simulink library "SimFly_Sensors"  (R2015b)
settings: Solver=VariableStepAuto  StartTime=0.0  StopTime=10.0  RelTol=1e-3
(part 2 of 2)

== matlab function SimFly_Sensors/GPS_UBX ==
  settings: updateMethod=DISCRETE  sampleTime=ubx_sample_time
  data: Ts output; lla output; flag_lla output; vel output; flag_vel output; sat output; alive output; time_delta output
function [Ts,lla,flag_lla,vel,flag_vel,sat,alive,time_delta] = ubx()
% Simulink Arduino Block Driver Library for Autocode Generation
 % 
 % This file is part of the Simulink Arduino Block Driver Library 
 % for Autocode Generation with Simulink
 %
 % This Library is free software: you can redistribute it and/or modify
 % it under the terms of the GNU General Public License as published by
 % the Free Software Foundation, either version 3 of the License, or
 % (at your option) any later version.
 %
 % This Library is distributed in the hope that it will be useful,
 % but WITHOUT ANY WARRANTY; without even the implied warranty of
 % MERCHANTABILITY or FITNESS FOR A PARTICULAR PURPOSE.  See the
 % GNU General Public License for more details.
 %
 % You should have received a copy of the GNU General Public License
 % along with this Library.  If not, see
 % <http://www.gnu.org/licenses/>.
 %
%
%PURPOSE: Driver for GPS UBX with hardware abstraction layer
%AUTHOR: Marcell Mocher
%DATE: 16.6.2016
%VERSION: 0.1 V Fist build
%Input: -
%Output:    Ts[1](uint32) =  GPS Millisecond from read
%           lla[3,1](double) =  Longitude Latitude Altitude in [deg] alt in [m]
%           flag_lla(boolean) = boolean for lla update 5Hz
%           vel[3,1](single) = ECEF X Y Z velocity m/s
%           flag_vel(boolean) = boolean for velocity update 5Hz
%           sat[1](uint8) = Number of visible satalites
%           alive[1](boolean) = Flag if UPX is alive and reads signals
%           with 5Hz update rate
%           time_delta(single) = time needed to execute funtion [us]
%Info: This drive requires function call triggered simuluink functions in
% order to work
%Requires:  [double] = getTime(),
%           [val_read] =  ardu_Serial1(uint8(called_function),uint32(baudrate),uint8(write_value));

persistent init_flag alive_flag state ck1 ck2 code id length idx data chk1...
    chk2 lastTime ack_count ack_flag lon lat alt gps_flag ecefXv ecefYv...
    ecefZv numSV vel_flag gps_num vel_num

if strcmp(coder.target, 'rtw'),
    
    
time_start = uint32(0);
time_start = coder.ceval('_get_time');

% Parameter from Mask!
baud = uint32(38400); % Standard Baudrate for UBX

% Init parameters

if isempty(init_flag)
    init_flag = 0;
    alive_flag = true;
    
    state = uint8(0);
    ck1 = uint64(0);
    ck2 = uint64(0);
    code = uint8(0);
    id = uint8(0);
    length = uint16(0);
    idx = uint16(0);
    data = uint8(zeros(512,1));
    chk1 = uint8(0);
    chk2 = uint8(0);
    lastTime = uint32(0);
    
    lon = double(0);
    lat = double(0);
    alt = double(0);
    ecefXv = single(0);
    ecefYv = single(0);
    ecefZv = single(0);
    numSV  = uint8(0);
    gps_num = uint8(0);
    vel_num = uint8(0);
    
    %Init Serial1 at 38000 baud
    coder.ceval('_serial_init',uint8(1),baud);
    
    ack_size= uint16(1); % Enter num of commands send!
    ack_flag = uint16(zeros(ack_size,1)); % Enter num of commands send!
    ack_count = uint16(1);
    
end

gps_flag = false;
vel_flag = false;

cc = uint8(0);
av = uint8(0);
av = coder.ceval('_serial_available',uint8(1));
if av > 0
    for i = 1:20
        cc = coder.ceval('_serial_read',uint8(1));
        switch state
            case 0 %wait for sync 1 (0xB5)
                ck1 = uint64(0);
                ck2 = uint64(0);
                if cc == 181 %0xB5
                    state = state + 1;
                end
            case 1 %wait for sync 2 (0x62)
                if cc == 98
                    state = state + 1;
                else
                    state = uint8(0);
                end
            case 2 %wait for class code
                code = cc;
                ck1 = ck1 + uint64(cc);
                if ck1 >= 256
                    ck1 = ck1 - uint64(256);
                end
                ck2 = ck2 + ck1;
                if ck2 >= 256
                    ck2 = ck2 - uint64(256);
                end
                state = state +1;
            case 3    % wait for Id
                id = cc;
                ck1 = ck1 + uint64(cc);
                if ck1 >= 256
                    ck1 = ck1 - uint64(256);
                end
                ck2 = ck2 + ck1;
                if ck2 >= 256
                    ck2 = ck2 - uint64(256);
                end
                state = state +1;
            case 4    % wait for length byte 1
                length = uint16(cc);
                ck1 = ck1 + uint64(cc);
                if ck1 >= 256
                    ck1 = ck1 - uint64(256);
                end
                ck2 = ck2 + ck1;
                if ck2 >= 256
                    ck2 = ck2 - uint64(256);
                end
                state = state +1;
            case 5   % wait for length byte 2
                val = uint16(cc);
                length = bitor(bitshift(val,8),length);
                ck1 = ck1 + uint64(cc);
                if ck1 >= 256
                    ck1 = ck1 - uint64(256);
                end
                ck2 = ck2 + ck1;
                if ck2 >= 256
                    ck2 = ck2 - uint64(256);
                end
                state = state + 1;
                idx = uint16(1);
                if length > 512
                    state = uint8(0);
                end
            case 6   % wait for <length> payload bytes
                data(idx) = cc;
                idx = idx + 1;
                ck1 = ck1 + uint64(cc);
                if ck1 >= 256
                    ck1 = ck1 - uint64(256);
                end
                ck2 = ck2 + ck1;
                if ck2 >= 256
                    ck2 = ck2 - uint64(256);
                end
                if (idx - 1 >= length)
                    state = state + 1;
                end
            case 7    % wait for checksum 1
                chk1 = cc;
                state = state + 1;
            case 8
                chk2 = cc;
                if (ck1 == chk1) && (ck2 == chk2)
                    switch code
                        case 1 %NAV-
                            lastTime = typecast(data(1:4),'uint32');
                            switch id
                                case 2 %NAV-POSLLH
                                    lon = double(typecast(data(5:8),'int32')) * 1e-7;
                                    lat = double(typecast(data(9:12),'int32')) * 1e-7;
                                    alt = double(typecast(data(13:16),'int32')) * 1e-3;
                                    gps_flag = true;
                                case 6 %NAV-SOL
                                    ecefXv = single(typecast(data(29:32),'int32')) * 1e-2; % m/s ECEF X velocity
                                    ecefYv = single(typecast(data(33:36),'int32')) * 1e-2; % m/s ECEF Y velocity
                                    ecefZv = single(typecast(data(37:40),'int32')) * 1e-2; % m/s ECEF Z velocity
                                    numSV  = typecast(data(48),'uint8'); % numSV
                                    vel_flag = true;
                            end
                        case 5 % ACK
                            switch id
                                case 0 % ACK-NAK Message Not Acknowledged
                                    if ack_count >= numel(ack_flag)
                                        ack_flag(ack_count) = false;
                                        ack_count = ack_count + 1;
                                    end
                                case 1 % ACK-NAK Message Acknowledged
                                    if ack_count >= numel(ack_flag)
                                        ack_flag(ack_count) = true;
                                        ack_count = ack_count + 1;
                                    end
                            end
                    end % End of switch (code)
                    state = uint8(0);
                else
                    state = uint8(0);
                end % End of checksum check
                
        end % End of switch (state)
        
    end % End for
    
end % End if

Ts = lastTime;
lla = [lon lat alt];
vel = [ecefXv ecefYv ecefZv];
sat = numSV;
flag_lla = gps_flag;
flag_vel = vel_flag;

if gps_flag == 0
    gps_num = gps_num + 1;
    if gps_num > 20
        alive_flag = false;
    end
else
    gps_num = uint8(0);
end

if vel_flag == 0
    vel_num = vel_num + 1;
    if vel_num > 20
        alive_flag = false;
    end
else
    vel_num = uint8(0);
end



% Only do readings if sensor is healthy
% if alive_flag == true
%
% end
alive = alive_flag;  %alive_flag;
time_end = uint32(0);
time_end = coder.ceval('_get_time');
time_delta = time_end - time_start;

else
Ts =  uint32(0);
lla = [0 0 0];
flag_lla = true;
vel = single([0 0 0]);
flag_vel = true;
sat = uint8(0);
alive = true;  %alive_flag;
time_delta = uint32(0);
end
end

== matlab function SimFly_Sensors/baro_alt ==
  settings: updateMethod=DISCRETE  sampleTime=alt_sample_time
  data: p input; baro_alt output; p0 parameter
function baro_alt  = baro_alt(p, p0)
% Simulink Arduino Block Driver Library for Autocode Generation
 % 
 % This file is part of the Simulink Arduino Block Driver Library 
 % for Autocode Generation with Simulink
 %
 % This Library is free software: you can redistribute it and/or modify
 % it under the terms of the GNU General Public License as published by
 % the Free Software Foundation, either version 3 of the License, or
 % (at your option) any later version.
 %
 % This Library is distributed in the hope that it will be useful,
 % but WITHOUT ANY WARRANTY; without even the implied warranty of
 % MERCHANTABILITY or FITNESS FOR A PARTICULAR PURPOSE.  See the
 % GNU General Public License for more details.
 %
 % You should have received a copy of the GNU General Public License
 % along with this Library.  If not, see
 % <http://www.gnu.org/licenses/>.
 %
%
%PURPOSE: Function to calculate the altitude from the pressure
%AUTHOR: Marcell Mocher
%DATE: 25.6.2016
%VERSION: 0.1 V Fist build
%Input: -
%Output:    alt[1](single) =  barometric altitude
%Info: 
%Requires:

%p0 = 1013.25;   % pressure at sea level in hPa

baro_alt = 44300*(1-(p/p0)^0.19); % barometric formula

== matlab function SimFly_Sensors/Gyro_L3GD20H ==
  settings: updateMethod=DISCRETE  sampleTime=l3gd20_sampletime
  data: gyro output; alive output; time_delta output; sD0Pin parameter; scaleValue parameter; freqValue parameter
function [gyro,alive,time_delta] = fcn(sD0Pin, scaleValue, freqValue)
% Simulink Arduino Block Driver Library for Autocode Generation
 % 
 % This file is part of the Simulink Arduino Block Driver Library 
 % for Autocode Generation with Simulink
 %
 % This Library is free software: you can redistribute it and/or modify
 % it under the terms of the GNU General Public License as published by
 % the Free Software Foundation, either version 3 of the License, or
 % (at your option) any later version.
 %
 % This Library is distributed in the hope that it will be useful,
 % but WITHOUT ANY WARRANTY; without even the implied warranty of
 % MERCHANTABILITY or FITNESS FOR A PARTICULAR PURPOSE.  See the
 % GNU General Public License for more details.
 %
 % You should have received a copy of the GNU General Public License
 % along with this Library.  If not, see
 % <http://www.gnu.org/licenses/>.
 %
%
%PURMPOSE: Driver for L3GD20H with hardware abstraction layer
%AUTHOR: Marcell Mocher
%DATE: 11.6.2016
%VERSION: 0.1V Fist build
%Input: -
%Output:    accel[3*1](single) = acceleration in X,Y,Z Axis [ms^-2]
%           mag[3*1](single) = magnetic field in X,Y,Z Axis [gauss]
%           alive(boolean) = boolean if sensor is alive
%           time_delta(single) = time needed to execute funtion [us]
%Info: This driver requires function call triggered simulink functions in
% order to work see requires
%Requires:  _get_time
%           _serial_init
%           _serial_print
%           _serial_write
%           _i2c_write_register
%           _i2c_read_register


persistent init_flag alive_flag sensibility L3GD20H_ADDR L3GD20_WHO_AM_I...
    L3GD20H_ID L3GD20_CTRL_REG1 L3GD20_CTRL_REG4

if strcmp(coder.target, 'rtw'),
    
    
    time_start = uint32(0);
    time_start = coder.ceval('_get_time');
    
    %Parameter from Mask!
    sd0 = sD0Pin;
    scale = scaleValue;
    freq = freqValue;
    
    if isempty(init_flag)
        init_flag = 0;
        alive_flag = false;
        gyro = single(zeros(3,1));
        L3GD20_WHO_AM_I = uint8(hex2dec('0F')); % Who AM I Register
        L3GD20H_ID = uint8(hex2dec('D7'));
        L3GD20_CTRL_REG1 = uint8(hex2dec('20'));
        L3GD20_CTRL_REG4 = uint8(hex2dec('23'));
        
        % Init functions
        coder.ceval('_i2c_init');
        
        % Assign MPU SA0 status
        if sd0 == true
            L3GD20H_ADDR = uint8(hex2dec('6B')); % High Address
        else
            L3GD20H_ADDR = uint8(hex2dec('6A')); % Low Address
        end
        
        %Check if sensor is connected
        val = uint8(zeros(6,1));
        coder.ceval('_i2c_read_register',L3GD20H_ADDR,L3GD20_WHO_AM_I,uint8(1),coder.ref(val));
        if  val(1) == L3GD20H_ID
            alive_flag = true;
        end
        
        % Start with normal mode -> all axes enabled
        % Datasheet = p36
        % Register 0x0F = 100Hz 12.5 Cutt of Hz
        % Register 0x1F = 100Hz 25 Cutt of Hz
        % Register 0x5F = 200Hz 0 Cutt of Hz
        % Register 0x4F = 200Hz 12.5 Cutt of Hz
        % Register 0x7F = 200Hz 70 Cutt of Hz
        % Register 0x8F = 400Hz 20   Cutt of Hz
        % Register 0xAF = 400Hz 50   Cutt of Hz
        % Register 0xBF = 400Hz 110   Cutt of Hz
        % Register 0xCF = 800Hz 30   Cutt of Hz
        % Register 0xFF = 800Hz 100   Cutt of Hz
        switch freq
            case 0 %100Hz 12.5 Cutt of Hz
                coder.ceval('_i2c_write_register',L3GD20H_ADDR,L3GD20_CTRL_REG1, uint8(hex2dec('0F')));
                
            case 1 %100Hz 25 Cutt of Hz
                coder.ceval('_i2c_write_register',L3GD20H_ADDR,L3GD20_CTRL_REG1, uint8(hex2dec('1F')));
            case 2 %200Hz 0 Cutt of Hz
                coder.ceval('_i2c_write_register',L3GD20H_ADDR,L3GD20_CTRL_REG1, uint8(hex2dec('5F')));
            case 3 %200Hz 12.5 Cutt of Hz
                coder.ceval('_i2c_write_register',L3GD20H_ADDR,L3GD20_CTRL_REG1, uint8(hex2dec('4F')));
            case 4 %200Hz 70 Cutt of Hz
                coder.ceval('_i2c_write_register',L3GD20H_ADDR,L3GD20_CTRL_REG1, uint8(hex2dec('7F')));
            case 5 %400Hz 20  Cutt of Hz
                coder.ceval('_i2c_write_register',L3GD20H_ADDR,L3GD20_CTRL_REG1, uint8(hex2dec('8F')));
            case 6 %400Hz 50   Cutt of Hz
                coder.ceval('_i2c_write_register',L3GD20H_ADDR,L3GD20_CTRL_REG1, uint8(hex2dec('AF')));
            case 7 %400Hz 110   Cutt of Hz
                coder.ceval('_i2c_write_register',L3GD20H_ADDR,L3GD20_CTRL_REG1, uint8(hex2dec('BF')));
            case 8 %800Hz 30   Cutt of Hz
                coder.ceval('_i2c_write_register',L3GD20H_ADDR,L3GD20_CTRL_REG1, uint8(hex2dec('CF')));
            case 9 %800Hz 100   Cutt of Hz
                coder.ceval('_i2c_write_register',L3GD20H_ADDR,L3GD20_CTRL_REG1, uint8(hex2dec('FF')));
        end
        
        % setting the Scale factor on register 4
        switch scale
            case 0 %L3GD20_SCALE_250
                sensibility = single(0.00875 * pi/180);
                coder.ceval('_i2c_write_register',L3GD20H_ADDR,L3GD20_CTRL_REG4, uint8(hex2dec('00')));
            case 1 %L3GD20_SCALE_500
                sensibility = single(0.0175 * pi/180);
                coder.ceval('_i2c_write_register',L3GD20H_ADDR,L3GD20_CTRL_REG4, uint8(hex2dec('10')));
            case 2 %L3GD20_SCALE_2000
                sensibility = single(0.070 * pi/180);
                coder.ceval('_i2c_write_register',L3GD20H_ADDR,L3GD20_CTRL_REG4, uint8(hex2dec('20')));
            otherwise
                sensibility = single(0.00875 * pi/180);
                coder.ceval('_i2c_write_register',L3GD20H_ADDR,L3GD20_CTRL_REG4, uint8(hex2dec('00')));
        end
        
    end
    
    % Read Gyro Register
    if alive_flag == true
        
        val = uint8(zeros(6,1));
        coder.ceval('_i2c_read_register',L3GD20H_ADDR,uint8(168),uint8(6),coder.ref(val));
        gyro(2) = single(typecast([val(1) val(2)],'int16'))* sensibility;
        gyro(1) = single(typecast([val(3) val(4)],'int16'))* sensibility;
        gyro(3) = -single(typecast([val(5) val(6)],'int16'))* sensibility;
    else
        
        gyro = single(zeros(3,1));
        
    end
    
    alive = alive_flag;
    time_end = uint32(0);
    time_end = coder.ceval('_get_time');
    time_delta = time_end - time_start;
else
    
    gyro = single(zeros(3,1));
    alive = true;
    time_delta = uint32(1);
end

== matlab function SimFly_Sensors/Baro_MS561101BA ==
  settings: updateMethod=DISCRETE  sampleTime=ms5611_sample_time
  data: pressure output; temp output; alive output; time_delta output; sD0Pin parameter; osrValue parameter
function [pressure,temp,alive,time_delta] = MS561101BA(  sD0Pin, osrValue)
% Simulink Arduino Block Driver Library for Autocode Generation
 % 
 % This file is part of the Simulink Arduino Block Driver Library 
 % for Autocode Generation with Simulink
 %
 % This Library is free software: you can redistribute it and/or modify
 % it under the terms of the GNU General Public License as published by
 % the Free Software Foundation, either version 3 of the License, or
 % (at your option) any later version.
 %
 % This Library is distributed in the hope that it will be useful,
 % but WITHOUT ANY WARRANTY; without even the implied warranty of
 % MERCHANTABILITY or FITNESS FOR A PARTICULAR PURPOSE.  See the
 % GNU General Public License for more details.
 %
 % You should have received a copy of the GNU General Public License
 % along with this Library.  If not, see
 % <http://www.gnu.org/licenses/>.
 %
%
%PURPOSE: Driver for MS561101BA with hardware abstraction layer
%AUTHOR: Marcell Mocher
%DATE: 10.6.2016
%VERSION: 0.1 V Fist build
%Input: -
%Output:    gyro[3*1](single) =  angular rates in X,Y,Z Axis [rad/s]
%           accel[3*1](single) = acceleration in X,Y,Z Axis [ms^-2]
%           alive(boolean) = boolean if sensor is alive
%           time_delta(single) = time needed to execute funtion [us]
%Info: This drive requires function call triggered simuluink functions in
% order to work
%Requires:  _get_time
%           _serial_init
%           _serial_print
%           _serial_write
%           _i2c_write_register
%           _i2c_read_register
%           _delay_us

persistent init_flag alive_flag delay_time osrc faccal MS5611_ADDR state...
    startTimeTemp startTimePress SENS OFF MS5611_D2 MS5611_D1 rawTemp...
    ms5611Temperature ms5611Pressure

if strcmp(coder.target, 'rtw'),
    
    time_start = uint32(0);
    time_start = coder.ceval('_get_time');
    
    % Parameter from Mask!
    sd0 =     sD0Pin;
    osr = osrValue;
    
    
    if isempty(init_flag)
        % Persistent values declaration
        init_flag = 0;
        faccal = uint16(zeros(6,1));
        state = uint8(0);
        startTimeTemp = uint32(0);
        startTimePress = uint32(0);
        SENS = int64(0);
        OFF = int64(0);
        rawTemp = uint32(0);
        ms5611Temperature = single(0);
        ms5611Pressure = single(0);
        
        MS5611_D1					= uint8(hex2dec('40'));		% registers
        MS5611_D2					= uint8(hex2dec('50'));		% registers
        
        MS5611_RESET				= uint8(hex2dec('1E'));		% registers
        MS5611_OSR_256 				= uint8(hex2dec('00'));		% Over Sampling Ratio constants
        MS5611_OSR_512 				= uint8(hex2dec('02'));		% Over Sampling Ratio constants
        MS5611_OSR_1024 			= uint8(hex2dec('04'));		% Over Sampling Ratio constants
        MS5611_OSR_2048 			= uint8(hex2dec('06'));		% Over Sampling Ratio constants
        MS5611_OSR_4096 			= uint8(hex2dec('08'));		% Over Sampling Ratio constants
        
        % Init funtions
        coder.ceval('_i2c_init');
        coder.ceval('_serial_init',uint32(250000));
        % Devices address
        if sd0 == true
            MS5611_ADDR = uint8(hex2dec('76')); % High
        else
            MS5611_ADDR = uint8(hex2dec('77')); % Low
        end
        
        % Reset device
        coder.ceval('_i2c_write_register',MS5611_ADDR,MS5611_RESET,uint8(0));
        
        % I have to wait here for 5ms!
        coder.ceval('_delay_us',uint32(5000));
        
        % Set oversampling rate
        switch osr
            case 0 % Sets the oversampling delay
                delay_time = uint32(1000); % microseconds sampling delay
                osrc = MS5611_OSR_256;
            case 1
                delay_time = uint32(2000);
                osrc = MS5611_OSR_512;
            case 2
                delay_time = uint32(3000);
                osrc = MS5611_OSR_1024;
            case 3
                delay_time = uint32(5000);
                osrc = MS5611_OSR_2048;
            case 4
                delay_time = uint32(10000);
                osrc = MS5611_OSR_4096;
            otherwise
                delay_time = uint32(1000);
                osrc = MS5611_OSR_256;
        end
        
        % Reads factory calibration and store it into object variables.
        
        for i = 1:6
            val = uint8(zeros(6,1));
            coder.ceval('_i2c_read_register',MS5611_ADDR,uint8(162) + (i-1) * 2,uint8(2),coder.ref(val));
            faccal(i) = typecast([val(2) val(1)],'uint16');
        end
        
        % sensor has no who am i register so i'll check if i got any
        % readings to see if the sensor is healthy
        if faccal(1) ~= 0
            alive_flag = true;
        else
            alive_flag = false;
        end
        
    end
    
    if alive_flag == true
        switch state
            case 0 % start temp reading
                coder.ceval('_i2c_write_register',MS5611_ADDR,MS5611_D2 + osrc,uint8(0));
                startTimeTemp = coder.ceval('_get_time');
                state = state + 1;
            case 1 % wait for 4.5ms and then read Raw Temperature
                time = uint32(0);
                time = coder.ceval('_get_time');
                if (time - startTimeTemp) > delay_time
                    %read raw temp
                    val = uint8(zeros(6,1));
                    coder.ceval('_i2c_read_register',MS5611_ADDR,uint8(0),uint8(3),coder.ref(val));
                    rawTemp = typecast([val(3),val(2),val(1),0],'uint32');
                    dT = int64(rawTemp - bitshift(uint32(faccal(5)),8));
                    OFF = bitshift(int64(faccal(2)),16) + bitshift(int64(faccal(4)) * dT,-7);
                    SENS = bitshift(int64(faccal(1)),15) + bitshift(int64(faccal(3)) * dT,-8);
                    TEMP = 2000 + bitshift((dT * int64(faccal(6))),-23);
                    ms5611Temperature = single(TEMP) * 0.01;
                    OFF2 = int64(0);
                    SENS2 = int64(0);
                    if (TEMP < 2000)
                        OFF2 = bitshift(5 * ((TEMP - 2000) * (TEMP - 2000)),-1);
                        SENS2 = bitshift(5 * ((TEMP - 2000) * (TEMP - 2000)),-2);
                    end
                    if (TEMP < -1500)
                        OFF2 = OFF2 + 7 * ((TEMP + 1500) * (TEMP + 1500));
                        SENS2 = SENS2 + bitshift(11 * ((TEMP + 1500) * (TEMP + 1500)),-1);
                    end
                    OFF = OFF - OFF2;
                    SENS = SENS - SENS2;
                    coder.ceval('_i2c_write_register',MS5611_ADDR,MS5611_D1 + osrc,uint8(0));% start press reading
                    startTimePress = coder.ceval('_get_time');
                    state = state + 1;
                end
            case 2 % wait for delayOversampling and then read Raw Temperature
                time = uint32(0);
                time = coder.ceval('_get_time');
                if (time - startTimePress) > delay_time
                    %read raw temp
                    val = uint8(zeros(6,1));
                    coder.ceval('_i2c_read_register',MS5611_ADDR,uint8(0),uint8(3),coder.ref(val));
                    rawPres = typecast([val(3),val(2),val(1),0],'uint32');
                    ms5611Pressure = single(bitshift(bitshift(int64(rawPres) * SENS,-21) - OFF,-15));
                    ms5611Pressure = ms5611Pressure * 0.01;
                    state = uint8(0);
                end
            otherwise
                state = uint8(0);
        end
    end
    
    temp = ms5611Temperature;
    pressure = ms5611Pressure;
    alive = alive_flag;
    
    time_end = uint32(0);
    time_end = coder.ceval('_get_time');
    time_delta = time_end - time_start;
    
    
    % Simulation mode
else
    pressure = single(1);
    temp = single(1);
    alive = true;
    time_delta = uint32(1);
    
end
end
